simulink model "Mpc"  (R2024b)
settings: Solver=VariableStepAuto  StartTime=0.0  StopTime=10  RelTol=1e-3
undefined symbols (not defined in the file or in its folder): sigbuilder_block
libraries: mpclib x1
settings Model: Creator=AA  LastModifiedBy=Marco
settings SolverCC: AlgebraicLoopSolver=TrustRegion
settings DataIOCC: ReturnWorkspaceOutputs=off
settings DebuggingCC: UnconnectedInputMsg=warning  UnconnectedOutputMsg=warning  UnconnectedLineMsg=warning  ArithmeticOperatorsInVariantConditions=warning
settings ModelReferenceCC: EnableRefExpFcnMdlSchedulingChecks=on
settings SFSimCC: SimUseLocalCustomCode=off  CustomCodeUndefinedFunction=UseInterfaceOnly
settings RTWCC: RTWUseLocalCustomCode=off  GPUComputeCapability=3.5

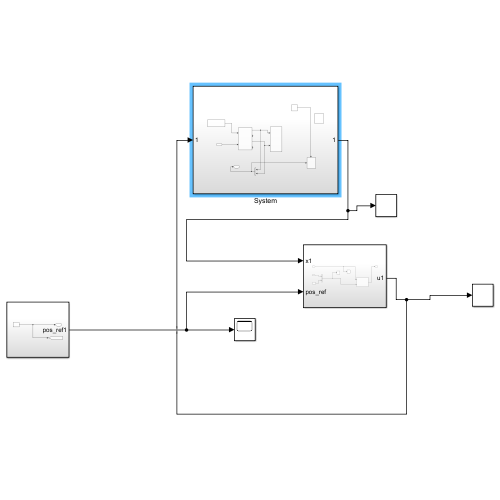
[thumbnail: Simulink's stored preview of the top-level diagram]
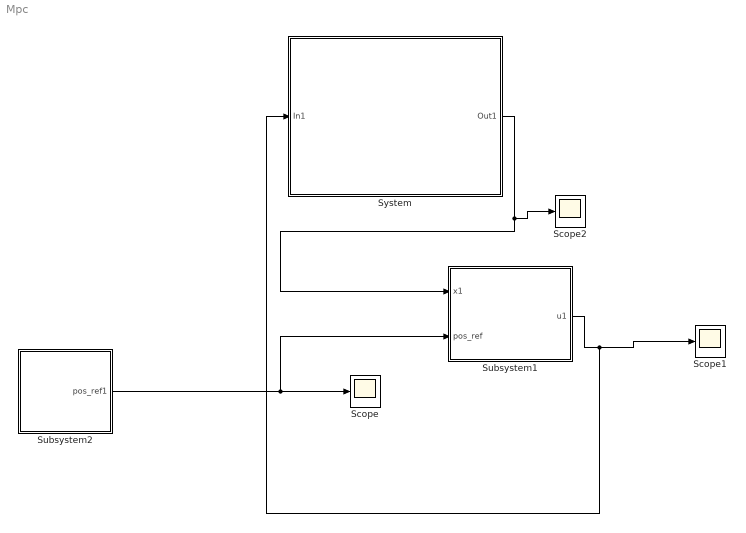
== system Mpc ==
  Scope : Scope
  Scope1 : Scope
  Scope2 : Scope
  Subsystem1 : Subsystem
  Subsystem2 : Subsystem
  System : Subsystem
  wires:
  System/1(Out1) -> Scope2/1, Subsystem1/1(x1)
  Subsystem2/1(pos_ref1) -> Scope/1, Subsystem1/2(pos_ref)
  Subsystem1/1(u1) -> System/1(In1), Scope1/1

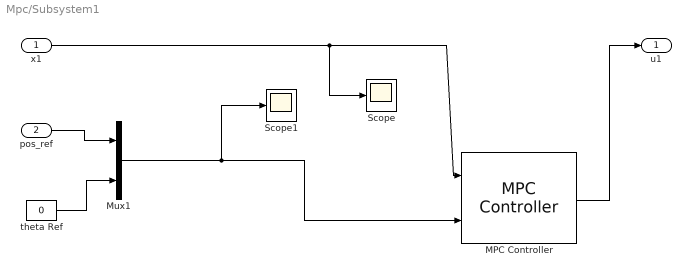
== system Mpc/Subsystem1 ==
  x1 : Inport
  pos_ref : Inport  Port=2
  MPC Controller : mpclib/MPC Controller  mpcobj=mpcobj  x0=[]  is_multiple=0  enable_value=0  return_u0=off  updateMPCinCallerWorkspace=on  md_inport=off  mv_inport=off  uref_inport=off  return_cost=off  return_mvseq=off  return_qpstatus=off  return_xseq=off  return_state=off  return_ovseq=off  state_inport=off  umin_inport=off  umax_inport=off  ymin_inport=off  ymax_inport=off  cc_inport=off  ywt_inport=off  uwt_inport=off  duwt_inport=off  rhoeps_inport=off  pm_inport=off  MaximumP=10  HorizonChoice=FixedHorizon  n_ts=0.01  n_p=50  n_mv=1  n_md=0  n_ud=1  n_mo=2  n_uo=0  BlockDataType=double  SampleTimeInherited=off  switch_inport=off
  Mux1 : Mux  Inputs=2
  Scope : Scope
  Scope1 : Scope
  theta Ref : Constant  Value=0
  u1 : Outport  VectorParamsAs1DForOutWhenUnconnected=off
  wires:
  pos_ref/1 -> Mux1/1
  MPC Controller/1 -> u1/1
  Mux1/1 -> Scope1/1, MPC Controller/2
  theta Ref/1 -> Mux1/2
  x1/1 -> Scope/1, MPC Controller/1

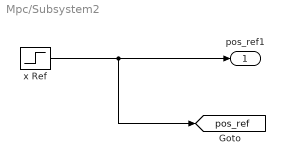
== system Mpc/Subsystem2 ==
  x Ref : Step  After=3  SampleTime=0
  pos_ref1 : Outport  VectorParamsAs1DForOutWhenUnconnected=off
  tag scope: pos_ref=global
  wires:
  x Ref/1 -> pos_ref1/1, [pos_ref]

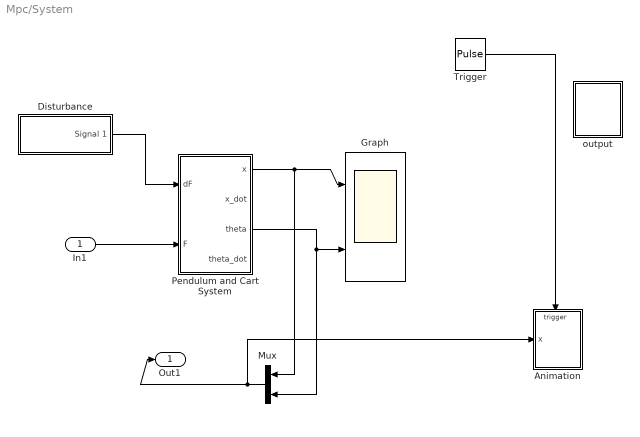
== system Mpc/System ==
  In1 : Inport
  Animation : Subsystem
  Disturbance : Subsystem  Tag=STV Subsys  LoadFcn=sigbuilder_block('load');  StartFcn=sigbuilder_block('start');  StopFcn=sigbuilder_block('stop');  ClipboardFcn=sigbuilder_block('clipboard');  mask(Sigbuilder block){tuvar=[0:10]}
      mask help: Simulink:masks:SigbuilderBlock_MD
      mask init:
      | if ~strcmp(get_param(bdroot(gcbh),'SimulationStatus'),'stopped') tuvar = sigbuilder_block('maskInit'); end
      settings: CopyFcn=sigbuilder_block('copy');  DeleteFcn=sigbuilder_block('delete');  ModelCloseFcn=sigbuilder_block('modelClose');  PreSaveFcn=sigbuilder_block('preSave');  PauseFcn=sigbuilder_block('pause');  ContinueFcn=sigbuilder_block('continue');  NameChangeFcn=sigbuilder_block('namechange');  OpenFcn=sigbuilder_block('open',[498 87 830.25 519 ]);  CloseFcn=sigbuilder_block('close');
      mask Display: plot(0, 0, 100, 100,[2, 2, 32, 32, 2], [68, 8, 8, 68, 68],[32, 2], [38, 38], [32, 19, 2],[53, 60, 44], [32, 17, 17, 2],[16, 16, 31, 31]);txt = getActiveGroup(gcbh);text(2, 100, txt,'verticalAlignment', 'top');
  Graph : Scope  NumInputPorts=2
  Mux : Mux  Inputs=2
  Pendulum and Cart System : Subsystem  mask{mCartPara=1, mPendPara=1, gPara=9.81, LPara=0.5, KdPara=10}
      mask prompts: mCartPara "Mass of Cart"; mPendPara "Mass of Pendulum"; gPara "Gravity"; LPara "Length of Pendulum"; KdPara "Friction coefficient of Cart"
      mask help: Pendulum and Cart System
      mask init:
      | mCart = str2double(get_param(gcb,'mCartPara'));
      | mPend = str2double(get_param(gcb,'mPendPara'));
      | g = str2double(get_param(gcb,'gPara'));
      | L = str2double(get_param(gcb,'LPara'));
      | Kd = str2double(get_param(gcb,'KdPara'));
  Trigger : DiscretePulseGenerator  PulseType=Time based  Period=0.1  PulseWidth=50
  output : Subsystem
  Out1 : Outport  VectorParamsAs1DForOutWhenUnconnected=off
  wires:
  Trigger/1 -> Animation/Trigger
  Pendulum and Cart System/1(x) -> Mux/1, Graph/1
  Pendulum and Cart System/3(theta) -> Graph/2, Mux/2
  In1/1 -> Pendulum and Cart System/2(F)
  Mux/1 -> Animation/1(x), Out1/1
  Disturbance/1(Signal 1) -> Pendulum and Cart System/1(dF)

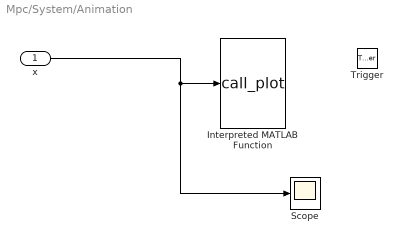
== system Mpc/System/Animation ==
  x : Inport
  Trigger : TriggerPort  VariantControl=(inherit)  PortDimensions=1
  Interpreted MATLAB Function : MATLABFcn  MATLABFcn=call_plot  OutputDimensions=0
  Scope : Scope
  wires:
  x/1 -> Scope/1, Interpreted MATLAB Function/1

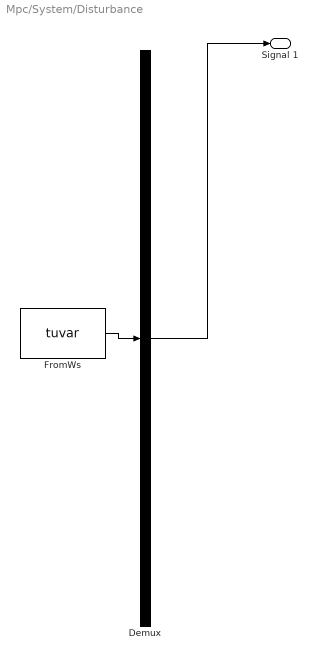
== system Mpc/System/Disturbance ==
  Demux : Demux  Tag=STV Demux  Outputs=1
      settings: DisplayOption=none
  FromWs : FromWorkspace  Tag=STV FromWs  VariableName=tuvar
      SigBuilderData=|
      | common.afterFinalStr = 'Extrapolate'
      | common.sampleTime = 0
      | dataSet.timeRange = [0 20]
      | dataSet.name = 'Group 1'
      | sbobj.Groups.Name = 'Group 1'
      | sbobj.Groups.Signals.Name = 'Signal 1'
      | sbobj.Groups.Signals.XData = [0 0.1 0.1 0.6 0.6 20]
      | sbobj.Groups.Signals.YData = [0 0 7 7 0 0]
      | sbobj.Groups.TimeRange = [0 20]
  Signal 1 : Outport  Tag=STV Outport
  wires:
  FromWs/1 -> Demux/1
  Demux/1 -> Signal 1/1

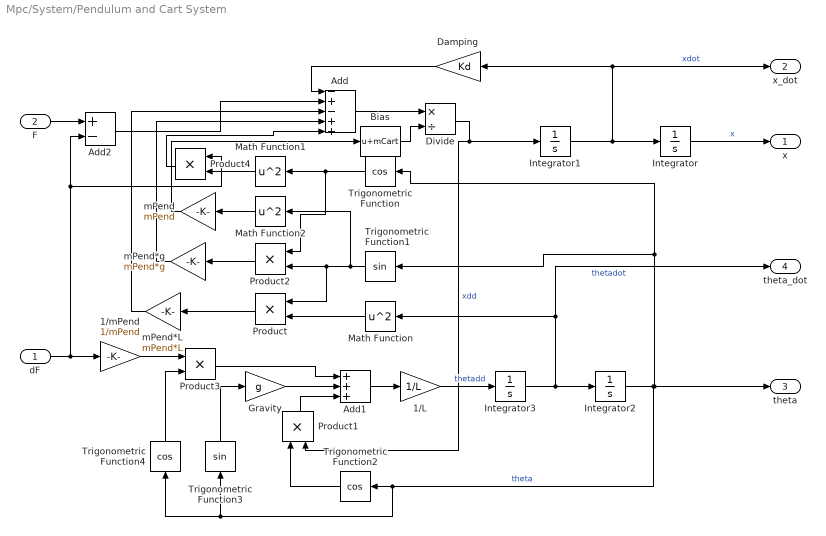
== system Mpc/System/Pendulum and Cart System ==
  dF : Inport
  F : Inport  Port=2
  1/L : Gain  Gain=1/L
  1/mPend : Gain  Gain=1/mPend
  Add : Sum  Inputs=-+-++
  Add1 : Sum  Inputs=+++
  Add2 : Sum  Inputs=+-
  Bias : Bias  Bias=mCart  SaturateOnIntegerOverflow=off
  Damping : Gain  Gain=Kd
  Divide : Product  Inputs=*/
  Gravity : Gain  Gain=g
  Integrator : Integrator  ContinuousStateAttributes='x'
  Integrator1 : Integrator  ContinuousStateAttributes='xdot'
  Integrator2 : Integrator  ContinuousStateAttributes='theta'
  Integrator3 : Integrator  ContinuousStateAttributes='thetadot'
  Math Function : Math  Operator=square  SignedPower=on
  Math Function1 : Math  Operator=square  SignedPower=on
  Math Function2 : Math  Operator=square  SignedPower=on
  Product{,1..4} (5 alike) : Product
  Trigonometric Function : Trigonometry  Operator=cos
  Trigonometric Function1 : Trigonometry
  Trigonometric Function2 : Trigonometry  Operator=cos
  Trigonometric Function3 : Trigonometry
  Trigonometric Function4 : Trigonometry  Operator=cos
  mPend : Gain  Gain=mPend
  mPend*L : Gain  Gain=mPend*L
  mPend*g : Gain  Gain=mPend*g
  x : Outport  VectorParamsAs1DForOutWhenUnconnected=off
  x_dot : Outport  Port=2  VectorParamsAs1DForOutWhenUnconnected=off
  theta : Outport  Port=3  VectorParamsAs1DForOutWhenUnconnected=off
  theta_dot : Outport  Port=4  VectorParamsAs1DForOutWhenUnconnected=off
  wires:
  mPend/1 -> Bias/1
  Bias/1 -> Divide/2
  Math Function2/1 -> mPend/1
  Product4/1 -> Add/5
  Math Function1/1 -> Product4/2
  mPend*g/1 -> Add/4
  Product1/1 -> Add1/3
  Math Function/1 -> Product/2
  1/L/1 -> Integrator3/1  "thetadd"
  dF/1 -> 1/mPend/1, Product4/1, Add2/2
  1/mPend/1 -> Product3/1
  Trigonometric Function4/1 -> Product3/2
  Damping/1 -> Add/1
  F/1 -> Add2/1
  Trigonometric Function3/1 -> Gravity/1
  Gravity/1 -> Add1/2
  Trigonometric Function/1 -> Math Function1/1, Product2/1
  Integrator3/1 -> Integrator2/1, Math Function/1, theta_dot/1  "thetadot"
  Integrator2/1 -> Trigonometric Function2/1, Trigonometric Function3/1, Trigonometric Function4/1, Trigonometric Function1/1, Trigonometric Function/1, theta/1  "theta"
  Product3/1 -> Add1/1
  Add/1 -> Divide/1
  Divide/1 -> Integrator1/1, Product1/2  "xdd"
  Trigonometric Function2/1 -> Product1/1
  Trigonometric Function1/1 -> Math Function2/1, Product/1, Product2/2
  Integrator/1 -> x/1  "x"
  Integrator1/1 -> Damping/1, x_dot/1, Integrator/1  "xdot"
  Product2/1 -> mPend*g/1
  Add1/1 -> 1/L/1
  Add2/1 -> Add/2
  mPend*L/1 -> Add/3
  Product/1 -> mPend*L/1

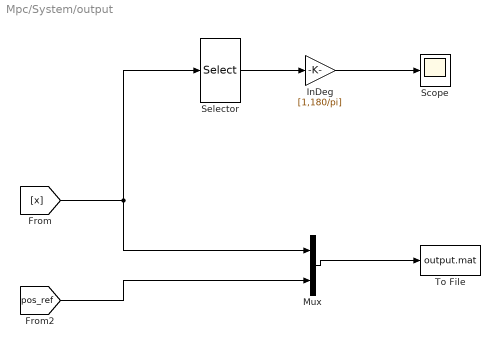
== system Mpc/System/output ==
  InDeg : Gain  Gain=[1,180/pi]
  Mux : Mux  Inputs=2
  Scope : Scope
  Selector : Selector  InputPortWidth=4  IndexOptions=Index vector (dialog)  Indices=[1:2]  OutputSizes=1
  To File : ToFile  Filename=output.mat  MatrixName=out  SaveFormat=Timeseries
  wires:
  [x] -> Mux/1, Selector/1
  InDeg/1 -> Scope/1
  Selector/1 -> InDeg/1
  Mux/1 -> To File/1
  [pos_ref] -> Mux/2
